simulink model "Assignment3"  (R2019a)
settings: Solver=FixedStepAuto  StartTime=0.0  StopTime=20  FixedStep=1  RelTol=1e-3
libraries: simulink x1
settings Model: Creator=Acer  LastModifiedBy=Acer

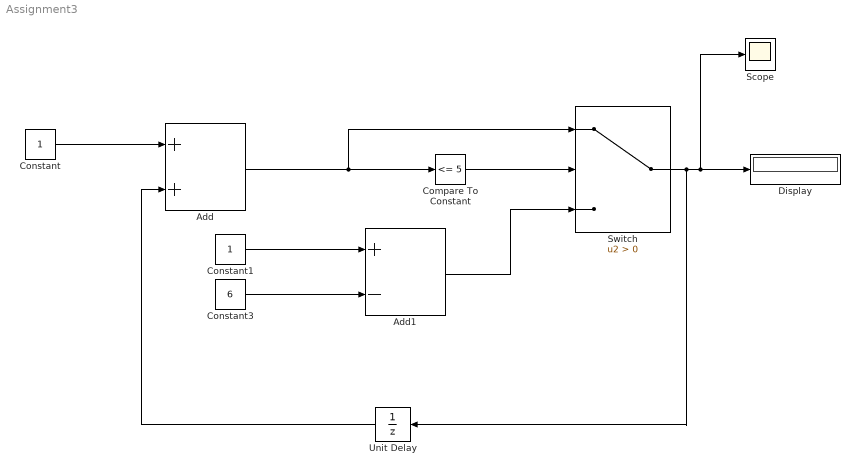
== system Assignment3 ==
  Add : Sum
  Add1 : Sum  Inputs=+-
  Compare To Constant : simulink/Logic and Bit Operations/Compare To Constant  relop=<=  const=5  OutDataTypeStr=boolean
  Constant : Constant
  Constant1 : Constant
  Constant3 : Constant  Value=6
  Display : Display
  Scope : Scope
  Switch : Switch  Criteria=u2 > Threshold
  Unit Delay : UnitDelay  SampleTime=-1  HasFrameUpgradeWarning=on
  wires:
  Constant/1 -> Add/1
  Add/1 -> Switch/1, Compare To Constant/1
  Compare To Constant/1 -> Switch/2
  Constant1/1 -> Add1/1
  Constant3/1 -> Add1/2
  Add1/1 -> Switch/3
  Switch/1 -> Unit Delay/1, Scope/1, Display/1
  Unit Delay/1 -> Add/2
